simulink model "randomNumber"  (R2015a)
settings: Solver=FixedStepDiscrete  SolverMode=SingleTasking  StartTime=0.0  StopTime=10.0  FixedStep=1e-3  RelTol=1e-3
libraries: mbed_targets_stm_disco_f407 x5, simulink x4
settings Model: Creator=Stuv  LastModifiedBy=Stuv
settings OptimizationCC: OptimizeModelRefInitCode=on  LifeSpan=1
settings HardwareCC: ProdLargestAtomicInteger=Long  ProdLargestAtomicFloat=Double  ProdEndianess=LittleEndian  ProdHWDeviceType=ARM Compatible->ARM Cortex
settings RTWCC: SystemTargetFile=mbed.tlc  TemplateMakefile=mbed.tmf  Description=Mbed Target (Embedded Target)  TargetLang=C++
settings CodeAppCC: IgnoreCustomStorageClasses=off
settings STFCustomTargetCC: CombineOutputUpdateFcns=on  SupportContinuousTime=off  SupportVariableSizeSignals=off  SystemTargetFile=mbed.tlc
settings ERTTargetCC: SupportContinuousTime=off  SupportVariableSizeSignals=off  ERTCustomFileTemplate=mbed_file_process.tlc

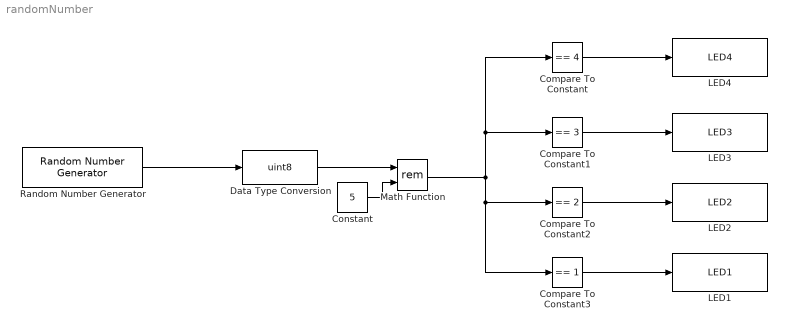
== system randomNumber ==
  Compare To Constant : simulink/Logic and Bit Operations/Compare To Constant  relop===  const=4  OutDataTypeStr=uint8
  Compare To Constant1 : simulink/Logic and Bit Operations/Compare To Constant  relop===  const=3  OutDataTypeStr=uint8
  Compare To Constant2 : simulink/Logic and Bit Operations/Compare To Constant  relop===  const=2  OutDataTypeStr=uint8
  Compare To Constant3 : simulink/Logic and Bit Operations/Compare To Constant  relop===  const=1  OutDataTypeStr=uint8
  Constant : Constant  Value=5  OutDataTypeStr=uint8
  Data Type Conversion : DataTypeConversion  OutDataTypeStr=uint8  ConvertRealWorld=Stored Integer (SI)
  LED1 : mbed_targets_stm_disco_f407/LED1  Parameter1=0
  LED2 : mbed_targets_stm_disco_f407/LED2  Parameter1=0
  LED3 : mbed_targets_stm_disco_f407/LED3  Parameter1=0
  LED4 : mbed_targets_stm_disco_f407/LED4  Parameter1=0
  Math Function : Math  Operator=rem  SaturateOnIntegerOverflow=on
  Random Number Generator : mbed_targets_stm_disco_f407/Random Number Generator  SampleTime=-1
  wires:
  Random Number Generator/1 -> Data Type Conversion/1
  Math Function/1 -> Compare To Constant1/1, Compare To Constant/1, Compare To Constant2/1, Compare To Constant3/1
  Data Type Conversion/1 -> Math Function/1
  Compare To Constant/1 -> LED4/1
  Compare To Constant1/1 -> LED3/1
  Compare To Constant2/1 -> LED2/1
  Compare To Constant3/1 -> LED1/1
  Constant/1 -> Math Function/2
